simulink model "Parcial_C"  (R2023b)
settings: Solver=ode4  StartTime=0.0  StopTime=100  FixedStep=0.0001  RelTol=1e-3
values from neighbouring files (symbols this model uses):
  ue = sin(x1e)    [Parcial.m]
  x1e = deg2rad(150)    [Parcial.m]
  x2e = 0    [Parcial.m]
libraries: cstblocks x1
settings Model: Creator=aghersin  LastModifiedBy=Usuario
settings SolverCC: AlgebraicLoopSolver=TrustRegion
settings DataIOCC: ReturnWorkspaceOutputs=off
settings OptimizationCC: LifeSpan=inf
settings DebuggingCC: UnconnectedInputMsg=warning  UnconnectedOutputMsg=warning  UnconnectedLineMsg=warning  SFExecutionAtInitializationDiag=none  ArithmeticOperatorsInVariantConditions=warning
settings ModelReferenceCC: EnableRefExpFcnMdlSchedulingChecks=on
settings SFSimCC: SimUseLocalCustomCode=off  CustomCodeUndefinedFunction=UseInterfaceOnly
settings RTWCC: RTWUseLocalCustomCode=off
settings CodeAppCC: StateflowObjectComments=on

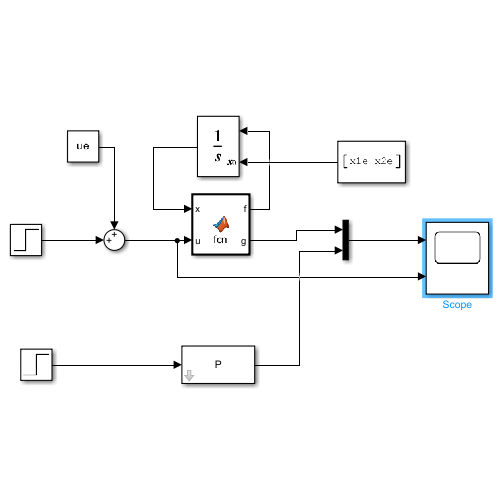
[thumbnail: Simulink's stored preview of the top-level diagram]
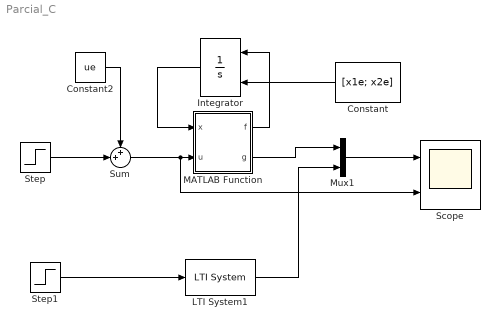
== system Parcial_C ==
  Constant : Constant  Value=[x1e; x2e]
  Constant2 : Constant  Value=ue
  Integrator : Integrator  InitialConditionSource=external
  LTI System1 : cstblocks/LTI System  sys=P  IC=[]  PadeOrder=0
  MATLAB Function : MATLAB Function  TreatAsAtomicUnit=on
  Mux1 : Mux  Inputs=2
  Scope : Scope  NumInputPorts=2
  Step : Step  After=0.2  SampleTime=0
  Step1 : Step  After=0.2  SampleTime=0
  Sum : Sum  Inputs=++|
  wires:
  Integrator/1 -> MATLAB Function/1(x)
  MATLAB Function/1(f) -> Integrator/1
  Constant/1 -> Integrator/2
  Constant2/1 -> Sum/1
  Sum/1 -> Scope/2, MATLAB Function/2(u)
  Step/1 -> Sum/2
  Step1/1 -> LTI System1/1
  Mux1/1 -> Scope/1
  MATLAB Function/2(g) -> Mux1/1
  LTI System1/1 -> Mux1/2

== matlab function Parcial_C/MATLAB Function ==
  data: x input; u input; f output; g output
function [f, g] = fcn(x,u)

f1 = x(2);
f2 = u - sin(x(1));
f = [f1; f2];

g = x(1);
